simulink model "Vehicle"  (R2024b)
settings: Solver=VariableStepAuto  StartTime=0.0  StopTime=50  RelTol=1e-3  EnableMultiTasking=on
libraries: fuzblock x1
settings Model: Creator=Atex  LastModifiedBy=Atea-wedi Rama
settings SolverCC: AlgebraicLoopSolver=TrustRegion
settings DataIOCC: ReturnWorkspaceOutputs=off
settings OptimizationCC: LifeSpan=inf
settings DebuggingCC: UnconnectedInputMsg=warning  UnconnectedOutputMsg=warning  UnconnectedLineMsg=warning  SFUnexpectedBacktrackingDiag=warning  SFNoUnconditionalDefaultTransitionDiag=warning  ArithmeticOperatorsInVariantConditions=warning
settings ModelReferenceCC: EnableRefExpFcnMdlSchedulingChecks=on
settings SFSimCC: SimUseLocalCustomCode=off  CustomCodeUndefinedFunction=UseInterfaceOnly
settings RTWCC: RTWUseLocalCustomCode=off  GPUComputeCapability=3.5
settings CodeAppCC: StateflowObjectComments=on
settings GRTTargetCC: TargetLangStandard=C89/C90 (ANSI)
settings ConfigComp: CovMetricSettings=dw  CovSaveCumulativeToWorkspaceVar=on  CovSaveSingleToWorkspaceVar=on  CovExternalEMLEnable=off

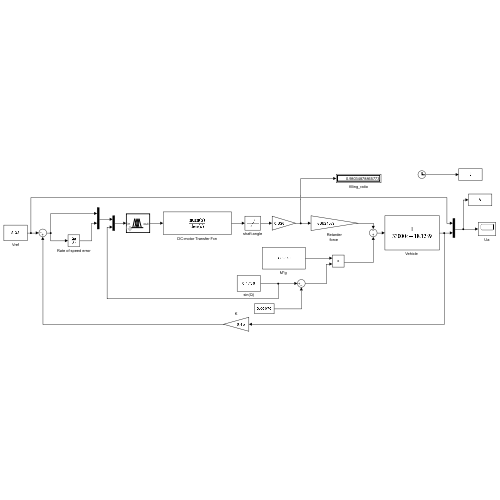
[thumbnail: Simulink's stored preview of the top-level diagram]
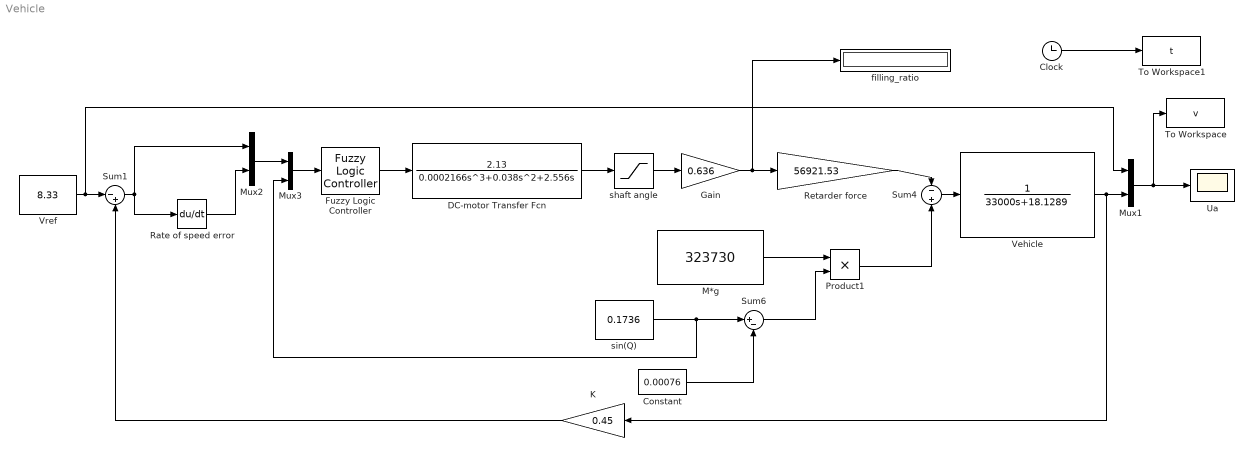
== system Vehicle ==
  Clock : Clock
  Constant : Constant  Value=0.00076
  DC-motor Transfer Fcn : TransferFcn  Numerator=[2.13]  Denominator=[0.0002166 0.038 2.556 0]
  Fuzzy Logic Controller : fuzblock/Fuzzy Logic  Controller  FIS=Fuzzy  OutputSampleNumber=101  DataType=double  FuzzifiedInputs=off  RuleFiringStrengths=off  RuleOutputs=off  AggregatedOutputs=off  SimulateUsing=Interpreted execution  OutOfRangeInputValueMessage=warning  NoRuleFiredMessage=warning  EmptyOutputFuzzySetMessage=warning
  Gain : Gain  Gain=0.636
  K : Gain  Gain=0.45
  "M*g " : Constant  Value=323730
  Mux1 : Mux  Inputs=2
  Mux2 : Mux  Inputs=2
  Mux3 : Mux  Inputs=2
  Product1 : Product
  Rate of speed error : Derivative
  "Retarder force " : Gain  Gain=56921.53
  Sum1 : Sum  Inputs=|-+
  Sum4 : Sum  Inputs=-+
  Sum6 : Sum  Inputs=|+-
  To Workspace : ToWorkspace  VariableName=v  SampleTime=-1
  To Workspace1 : ToWorkspace  VariableName=t  SampleTime=-1
  Ua : Scope
  "Vehicle " : TransferFcn  Denominator=[33000 18.1289]
  Vref : Constant  Value=8.33
  filling_ratio : Display
  shaft angle : Saturate  UpperLimit=pi/2  LowerLimit=-pi/2
  sin(Q) : Constant  Value=0.1736
  wires:
  Vref/1 -> Sum1/1, Mux1/1
  Product1/1 -> Sum4/2
  "M*g "/1 -> Product1/1
  Sum6/1 -> Product1/2
  Constant/1 -> Sum6/2
  Sum4/1 -> "Vehicle "/1
  Mux2/1 -> Mux3/1
  Mux3/1 -> Fuzzy Logic Controller/1
  Mux1/1 -> To Workspace/1, Ua/1
  "Retarder force "/1 -> Sum4/1
  shaft angle/1 -> Gain/1
  DC-motor Transfer Fcn/1 -> shaft angle/1
  Rate of speed error/1 -> Mux2/2
  "Vehicle "/1 -> Mux1/2, K/1
  K/1 -> Sum1/2
  Clock/1 -> To Workspace1/1
  Fuzzy Logic Controller/1 -> DC-motor Transfer Fcn/1
  sin(Q)/1 -> Mux3/2, Sum6/1
  Sum1/1 -> Rate of speed error/1, Mux2/1
  Gain/1 -> filling_ratio/1, "Retarder force "/1
